simulink model "incubator_sim"  (R2023a)
settings: Solver=VariableStepAuto  StartTime=0.0  StopTime=3600  RelTol=1e-3
values from neighbouring files (symbols this model uses):
  A_hum = L_hum*L_hum    (= 0.01)    [incubator.m]
  A_tot = 1.5112    [incubator.m]
  Acv = 0.9 * Sa    (= 0.163689221901)    [incubator.m]
  Anet = Amat - As    (= 0.1872)    [incubator.m]
  Ar = 0.555 * Sa    (= 0.100941686839)    [incubator.m]
  As = 0.36*0.15    (= 0.054)    [incubator.m]
  Awi = 1.2    [incubator.m]
  bf = 0.18*60 / 1000    (= 0.0108)    [incubator.m]
  cp_b = 3770    [incubator.m]
  cp_co = 3470    [incubator.m]
  cpa = 1005    [incubator.m]
  cpa_skin = 3400    [incubator.m]
  cpm = 1500    [incubator.m]
  cpw = 4e7    (= 40000000)    [incubator.m]
  eps_s = 0.97    [incubator.m]
  epsilon_w = 0.9    [incubator.m]
  Evap = 0.15e-9    (= 1.5e-10)    [incubator.m]
  h_m_hum = (D_hum / L_hum) * Sh_hum    (= 3.61503807077e-07)    [incubator.m]
  hacv = 20    [incubator.m]
  hf_g = 2.343e6    (= 2343000)    [incubator.m]
  hfg = 2.257e6    (= 2257000)    [incubator.m]
  hscv = (Nu * Ka) / Dsph    (= 0.464725290588)    [incubator.m]
  IV = 3.3e-6    (= 3.3e-06)    [incubator.m]
  K_c = 0.6    [incubator.m]
  Kmat = 0.07    [incubator.m]
  m = 2.46    [incubator.m]
  maire = 0.15    [incubator.m]
  mco = m_co    (= 1.41420774897)    [incubator.m]
  mdot_a = rho_a * A_entrada * v_max    (= 0.0036)    [incubator.m]
  ms = th_s * rho_s * Sa    (= 1.04579225103)    [incubator.m]
  mw = rho_w * th_w * Awi    (= 12.72)    [incubator.m]
  P_atm = 101325    [incubator.m]
  Qmet = mrst*Sa    (= 5.94999408995)    [incubator.m]
  R_hum = 461.5    [incubator.m]
  rho_a = 1.2    [incubator.m]
  rho_bl = 1060    [incubator.m]
  rho_c = 1050    [incubator.m]
  rho_w = 1060    [incubator.m]
  Sa = m^0.75/10.8    (= 0.181876913223)    [incubator.m]
  sigma = 5.670e-8    (= 5.67e-08)    [incubator.m]
  thm = 0.04    [incubator.m]
  V_aire = maire/rho_a    (= 0.125)    [incubator.m]
  Vb = m*100e-6    (= 0.000246)    [incubator.m]
  Wex = 44e-6/1.184e-3    (= 0.0371621621622)    [incubator.m]
undefined symbols (not defined in the file or in its folder): Qh
settings Model: Creator=ACER  LastModifiedBy=ACER

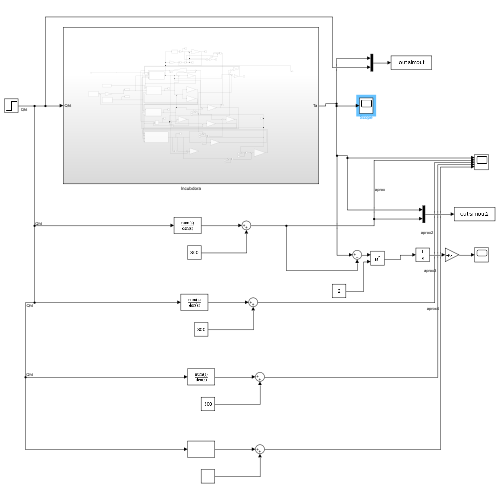
[thumbnail: Simulink's stored preview of the top-level diagram]
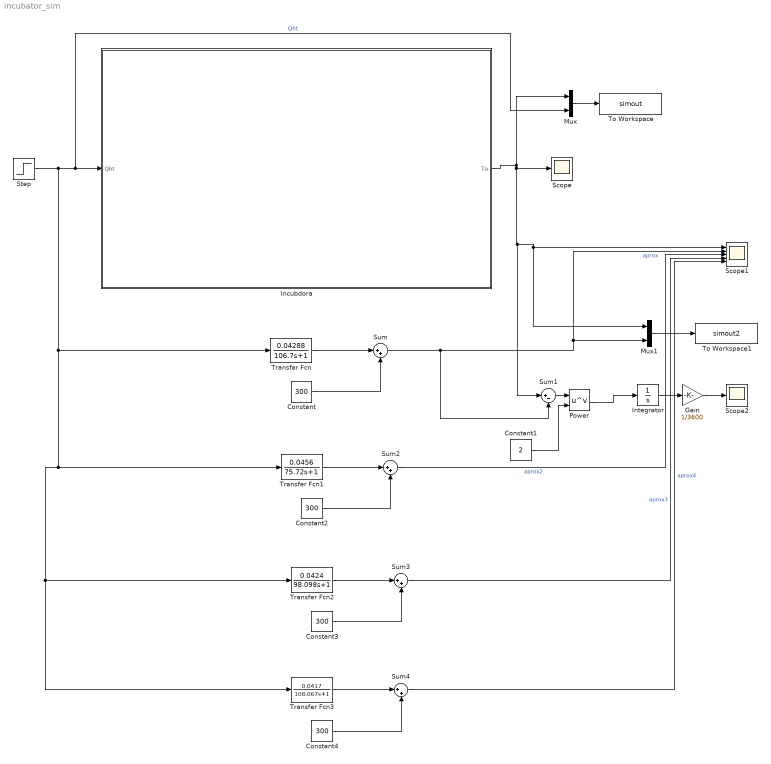
== system incubator_sim ==
  Constant{,2..4} (4 alike) : Constant  Value=300
  Constant1 : Constant  Value=2
  Gain : Gain  Gain=1/3600
  Incubdora : Subsystem
  Integrator : Integrator
  Mux : Mux  Inputs=2
  Mux1 : Mux  Inputs=2
  Power : Math  Operator=pow
  Scope : Scope
  Scope1 : Scope  NumInputPorts=5
  Scope2 : Scope
  Step : Step  Time=0  After=Qh  SampleTime=0
  Sum{,2..4} (4 alike) : Sum  Inputs=|++
  Sum1 : Sum  Inputs=|+-
  To Workspace : ToWorkspace  VariableName=simout  SaveFormat=Timeseries  SampleTime=-1
  To Workspace1 : ToWorkspace  VariableName=simout2  SaveFormat=Timeseries  SampleTime=-1
  Transfer Fcn : TransferFcn  Numerator=[0.04288]  Denominator=[106.7 1]
  Transfer Fcn1 : TransferFcn  Numerator=[0.0456]  Denominator=[75.72 1]
  Transfer Fcn2 : TransferFcn  Numerator=[ 0.0424]  Denominator=[98.098 1]
  Transfer Fcn3 : TransferFcn  Numerator=[0.0417]  Denominator=[108.067 1]
  wires:
  Incubdora/1(Ta) -> Sum1/1, Mux1/1, Scope1/1, Scope/1, Mux/1
  Mux/1 -> To Workspace/1
  Transfer Fcn/1 -> Sum/1
  Sum/1 -> Sum1/2, Mux1/2, Scope1/2  "aprox"
  Constant/1 -> Sum/2
  Mux1/1 -> To Workspace1/1
  Integrator/1 -> Gain/1
  Sum1/1 -> Power/1
  Power/1 -> Integrator/1
  Constant1/1 -> Power/2
  Gain/1 -> Scope2/1
  Constant2/1 -> Sum2/2
  Sum2/1 -> Scope1/3  "aprox2"
  Transfer Fcn1/1 -> Sum2/1
  Sum3/1 -> Scope1/4  "aprox3"
  Constant3/1 -> Sum3/2
  Transfer Fcn2/1 -> Sum3/1
  Sum4/1 -> Scope1/5  "aprox4"
  Step/1 -> Transfer Fcn1/1, Transfer Fcn3/1, Transfer Fcn2/1, Transfer Fcn/1, Mux/2, Incubdora/1(Qht)  "Qht"
  Constant4/1 -> Sum4/2
  Transfer Fcn3/1 -> Sum4/1

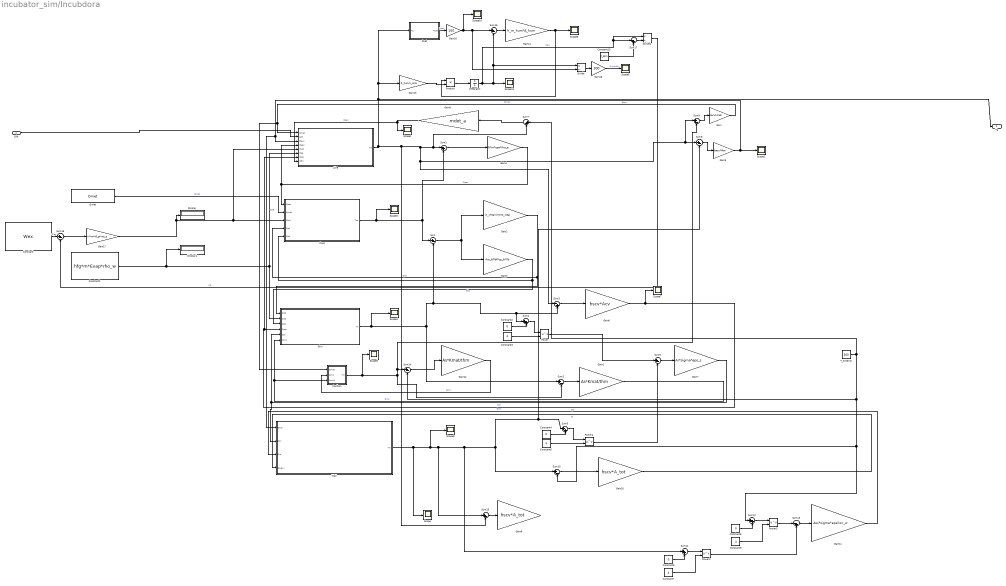
== system incubator_sim/Incubdora ==
  Qht : Inport
  Aire : Subsystem
  Coclhon : Subsystem
  Constant : Constant  Value=Wex
  Constant1 : Constant  Value=hfg*m*Evap*rho_w
  Constant10 : Constant  Value=P_atm
  Constant{2,4,6,8} (4 alike) : Constant  Value=0
  Constant{3,5,7,9} (4 alike) : Constant  Value=4
  Core : Subsystem
  Display : Display
  Display1 : Display
  Divide : Product  Inputs=*/
  Divide1 : Product  Inputs=*/
  Gain : Gain  Gain=hacv*Anet
  Gain1 : Gain  Gain=As*Kmat/thm
  Gain10 : Gain  Gain=hscv*A_tot
  Gain11 : Gain  Gain=Awi*sigma*epsilon_w
  Gain12 : Gain  Gain=As*Kmat/thm
  Gain13 : Gain  Gain=R_hum/V_aire
  Gain14 : Gain  Gain=h_m_hum*A_hum
  Gain15 : Gain  Gain=100
  Gain16 : Gain  Gain=100
  Gain17 : Gain  Gain=IV*m*hf_g*rho_a
  Gain2 : Gain  Gain=(K_c*Sa)/(m/rho_c/Sa)
  Gain3 : Gain  Gain=rho_bl*bf*cp_b*Vb
  Gain4 : Gain  Gain=IV*m*cpa*rho_a
  Gain5 : Gain  Gain=hacv*Awi
  Gain6 : Gain  Gain=hscv*Acv
  Gain7 : Gain  Gain=Ar*sigma*eps_s
  Gain8 : Gain  Gain=hscv*A_tot
  Gain9 : Gain  Gain=mdot_a
  Integrator : Integrator
  Power{,1..3} (4 alike) : Math  Operator=pow
  Product : Product
  Psat : Subsystem
  Qmet : Constant  Value=Qmet
  Scope{,1..11} (12 alike) : Scope
  Skin : Subsystem
  Sum{,2,6..10,14..16,18} (11 alike) : Sum  Inputs=|+-
  Sum{1,3,13,17} (4 alike) : Sum  Inputs=|-+
  Sum{4..5,11..12} (4 alike) : Sum  Inputs=|++
  T_exterior : Constant  Value=300
  Wall : Subsystem
  Ta : Outport
  wires:
  Gain/1 -> Aire/1(Qmat), Coclhon/1(Qmat)  "Qmat"
  Gain5/1 -> Scope2/1, Wall/1(Qacv), Aire/3(Qacv)  "Qacv"
  Power/1 -> Sum6/1
  Gain2/1 -> Skin/1(Qcd), Core/4(Qcd)  "Qcd"
  Sum1/1 -> Gain4/1
  Constant3/1 -> Power/2
  Aire/1(Ta) -> Ta/1, Psat/1(Ta), Gain13/1, Sum15/2, Sum9/1, Sum8/1, Sum3/1, Sum7/2, Sum1/1
  Qmet/1 -> Core/2(Qmet)  "Qmet"
  Power1/1 -> Sum6/2
  Sum4/1 -> Power/1
  Sum3/1 -> Gain6/1
  Sum14/1 -> Gain12/1
  Sum5/1 -> Power1/1
  Constant2/1 -> Sum4/2
  Gain7/1 -> Wall/2(Qsr), Skin/5(Qsr)  "Qsr"
  Gain4/1 -> Aire/4(Qsen), Core/1(Qsen)  "Qsen"
  Constant1/1 -> Display1/1, Skin/2(Qse), Aire/6(Qse)  "Qse"
  Sum/1 -> Gain3/1, Gain2/1
  Gain11/1 -> Wall/3(Qro)  "Qro"
  Sum13/1 -> Gain11/1
  Constant8/1 -> Sum12/2
  Gain1/1 -> Skin/6(Qmc), Coclhon/3(Qmc1)  "Qmc"
  Core/1(Tco) -> Scope3/1, Sum1/2, Sum/1
  Constant4/1 -> Sum5/2
  Wall/1(Tw) -> Scope/1, Sum10/1, Sum8/2, Sum5/1, Sum11/1, Sum15/1, Scope5/1
  Skin/1(Ts) -> Scope4/1, Sum4/1, Sum3/2, Sum/2, Sum2/1
  Constant5/1 -> Power1/2
  Constant6/1 -> Sum11/2
  Sum2/1 -> Gain1/1
  Gain6/1 -> Scope7/1, Aire/7(Qscv), Skin/4(Qscv)  "Qscv"
  Gain3/1 -> Skin/3(Qbc), Core/5(Qbc)  "Qbc"
  Sum8/1 -> Gain5/1
  Power2/1 -> Sum13/2
  T_exterior/1 -> Sum14/2, Sum10/2, Sum12/1, Sum7/1
  Sum12/1 -> Power3/1
  Constant7/1 -> Power2/2
  Constant9/1 -> Power3/2
  Sum6/1 -> Gain7/1
  Sum9/1 -> Gain/1
  Sum11/1 -> Power2/1
  Power3/1 -> Sum13/1
  Coclhon/1(Tm) -> Scope6/1, Sum2/2, Sum14/1, Sum9/2
  Qht/1 -> Aire/2(Qht)
  Gain12/1 -> Coclhon/2(Qmc)  "Qmc"
  Sum7/1 -> Gain9/1
  Gain9/1 -> Scope1/1, Aire/8(Qfm)  "Qsen"
  Sum15/1 -> Gain8/1
  Gain10/1 -> Wall/4(Qoenv)  "Qi"
  Sum10/1 -> Gain10/1
  Psat/1(Psat) -> Gain16/1  "Psat"
  Integrator/1 -> Divide1/1, Sum17/1, Scope11/1, Divide/1, Sum16/2  "Pair"
  Sum16/1 -> Gain14/1
  Gain13/1 -> Product/2
  Product/1 -> Integrator/1
  Gain14/1 -> Scope9/1, Product/1
  Divide/1 -> Gain15/1
  Gain15/1 -> Scope8/1  "Humidity"
  Gain16/1 -> Scope10/1, Divide/2, Sum16/1
  Constant10/1 -> Sum17/2
  Sum17/1 -> Divide1/2
  Divide1/1 -> Sum18/2  "wa"
  Constant/1 -> Sum18/1  "Qlat"
  Sum18/1 -> Gain17/1
  Gain17/1 -> Aire/5(Qlat), Core/3(Qlat), Display/1

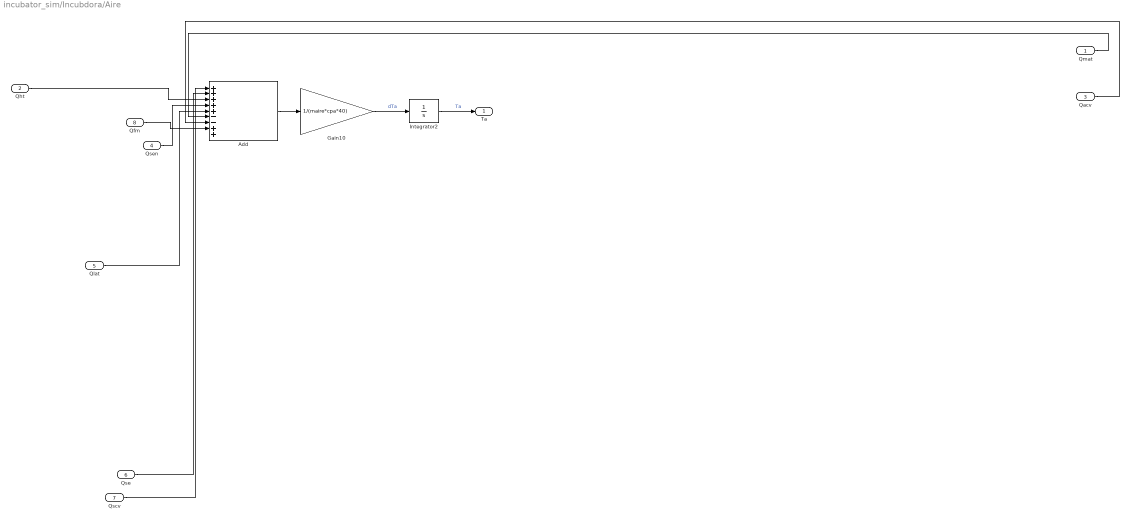
== system incubator_sim/Incubdora/Aire ==
  Qmat : Inport
  Qht : Inport  Port=2
  Qacv : Inport  Port=3
  Qsen : Inport  Port=4
  Qlat : Inport  Port=5
  Qse : Inport  Port=6
  Qscv : Inport  Port=7
  Qfm : Inport  Port=8
  Add : Sum  Inputs=+++++--++
  Gain10 : Gain  Gain=1/(maire*cpa*40)
  Integrator2 : Integrator  InitialCondition=300
  Ta : Outport
  wires:
  Qse/1 -> Add/2
  Qsen/1 -> Add/4
  Qlat/1 -> Add/5
  Add/1 -> Gain10/1
  Integrator2/1 -> Ta/1  "Ta"
  Gain10/1 -> Integrator2/1  "dTa"
  Qscv/1 -> Add/1
  Qacv/1 -> Add/7
  Qmat/1 -> Add/6
  Qht/1 -> Add/3
  Qfm/1 -> Add/8

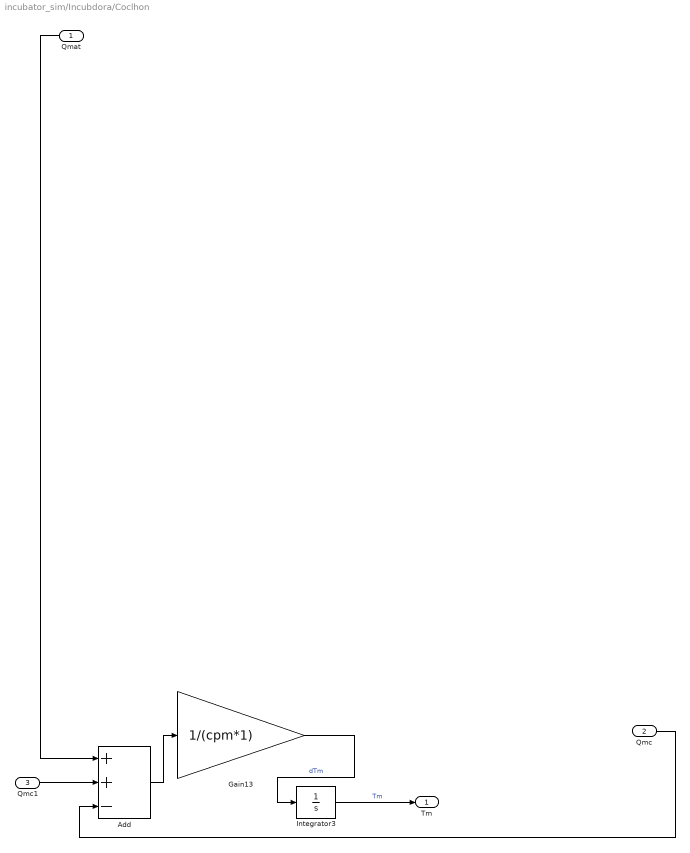
== system incubator_sim/Incubdora/Coclhon ==
  Qmat : Inport
  Qmc : Inport  Port=2
  Qmc1 : Inport  Port=3
  Add : Sum  Inputs=++-
  Gain13 : Gain  Gain=1/(cpm*1)
  Integrator3 : Integrator  InitialCondition=300
  Tm : Outport
  wires:
  Integrator3/1 -> Tm/1  "Tm"
  Add/1 -> Gain13/1
  Gain13/1 -> Integrator3/1  "dTm"
  Qmc/1 -> Add/3
  Qmat/1 -> Add/1
  Qmc1/1 -> Add/2

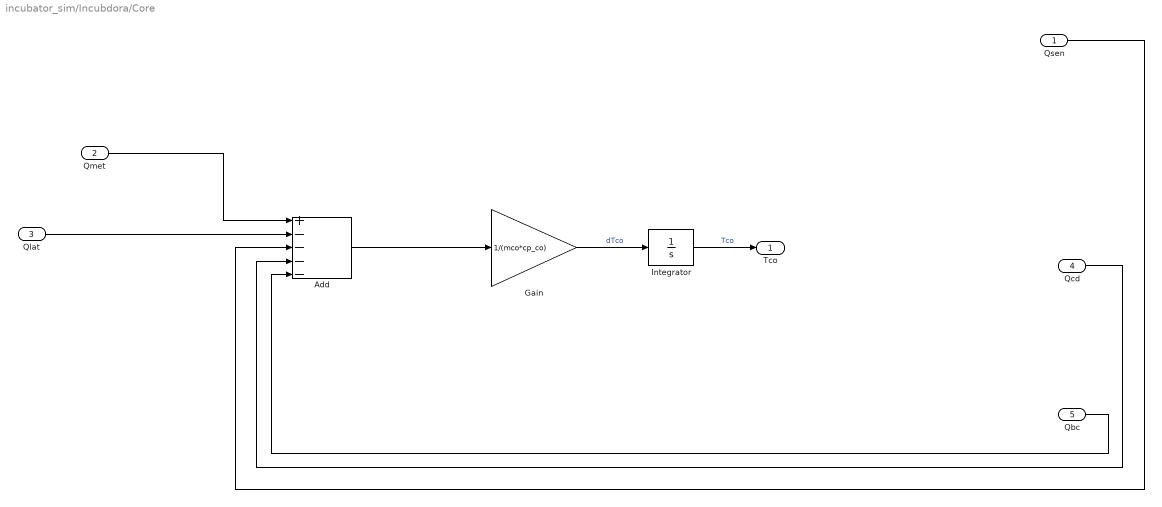
== system incubator_sim/Incubdora/Core ==
  Qsen : Inport
  Qmet : Inport  Port=2
  Qlat : Inport  Port=3
  Qcd : Inport  Port=4
  Qbc : Inport  Port=5
  Add : Sum  Inputs=+----
  Gain : Gain  Gain=1/(mco*cp_co)
  Integrator : Integrator  InitialCondition=308
  Tco : Outport
  wires:
  Qlat/1 -> Add/2
  Gain/1 -> Integrator/1  "dTco"
  Qbc/1 -> Add/5
  Qcd/1 -> Add/4
  Integrator/1 -> Tco/1  "Tco"
  Add/1 -> Gain/1
  Qmet/1 -> Add/1
  Qsen/1 -> Add/3

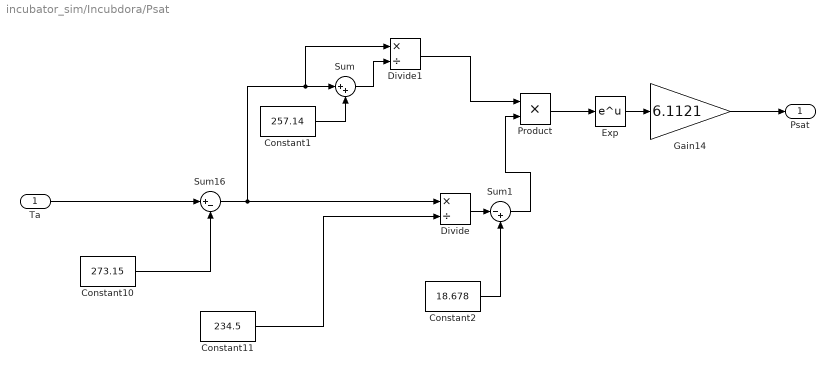
== system incubator_sim/Incubdora/Psat ==
  Ta : Inport
  Constant1 : Constant  Value=257.14
  Constant10 : Constant  Value=273.15
  Constant11 : Constant  Value=234.5
  Constant2 : Constant  Value=18.678
  Divide : Product  Inputs=*/
  Divide1 : Product  Inputs=*/
  Exp : Math
  Gain14 : Gain  Gain=6.1121
  Product : Product
  Sum : Sum  Inputs=|++
  Sum1 : Sum  Inputs=|-+
  Sum16 : Sum  Inputs=|+-
  Psat : Outport
  wires:
  Constant11/1 -> Divide/2
  Gain14/1 -> Psat/1
  Constant10/1 -> Sum16/2
  Ta/1 -> Sum16/1
  Sum16/1 -> Divide1/1, Sum/1, Divide/1
  Constant1/1 -> Sum/2
  Sum/1 -> Divide1/2
  Divide1/1 -> Product/1
  Constant2/1 -> Sum1/2
  Product/1 -> Exp/1
  Exp/1 -> Gain14/1
  Divide/1 -> Sum1/1
  Sum1/1 -> Product/2

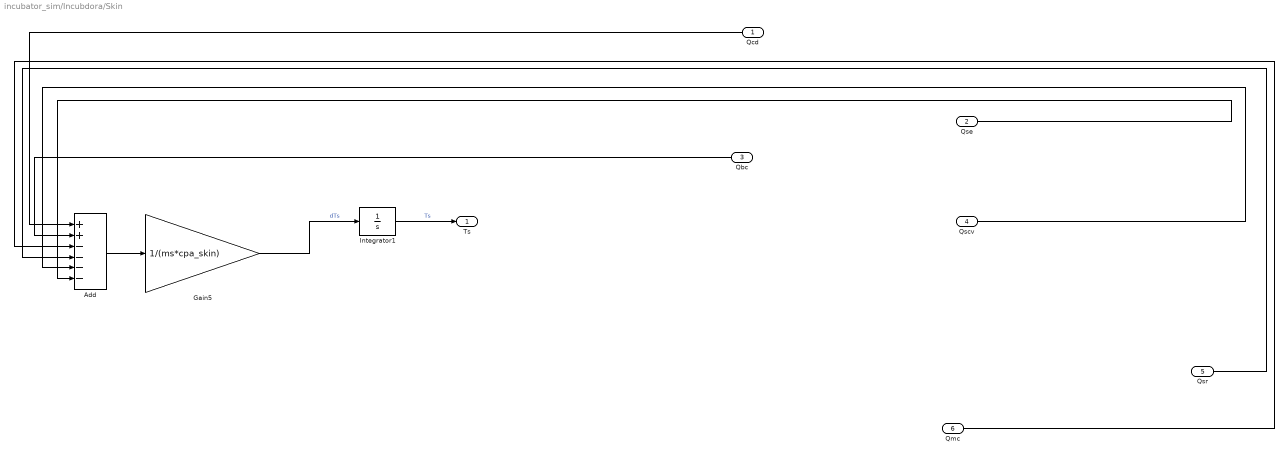
== system incubator_sim/Incubdora/Skin ==
  Qcd : Inport
  Qse : Inport  Port=2
  Qbc : Inport  Port=3
  Qscv : Inport  Port=4
  Qsr : Inport  Port=5
  Qmc : Inport  Port=6
  Add : Sum  Inputs=++----
  Gain5 : Gain  Gain=1/(ms*cpa_skin)
  Integrator1 : Integrator  InitialCondition=308
  Ts : Outport
  wires:
  Qbc/1 -> Add/2
  Qscv/1 -> Add/5
  Add/1 -> Gain5/1
  Gain5/1 -> Integrator1/1  "dTs"
  Qse/1 -> Add/6
  Qmc/1 -> Add/3
  Qsr/1 -> Add/4
  Integrator1/1 -> Ts/1  "Ts"
  Qcd/1 -> Add/1

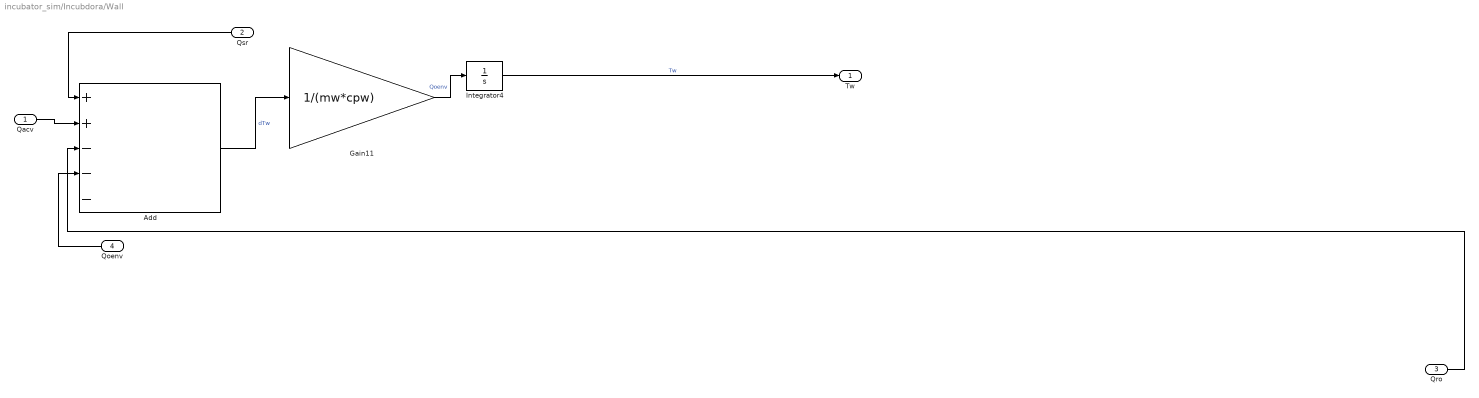
== system incubator_sim/Incubdora/Wall ==
  Qacv : Inport
  Qsr : Inport  Port=2
  Qro : Inport  Port=3
  Qoenv : Inport  Port=4
  Add : Sum  Inputs=++---
  Gain11 : Gain  Gain=1/(mw*cpw)
  Integrator4 : Integrator  InitialCondition=300
  Tw : Outport
  wires:
  Add/1 -> Gain11/1  "dTw"
  Qsr/1 -> Add/1
  Qacv/1 -> Add/2
  Gain11/1 -> Integrator4/1  "Qoenv"
  Qro/1 -> Add/3
  Integrator4/1 -> Tw/1  "Tw"
  Qoenv/1 -> Add/4
